simulink model "Boat_Sim"  (R2017a)
settings: Solver=VariableStepAuto  StartTime=0.0  StopTime=10.0  RelTol=1e-3
values from neighbouring files (symbols this model uses):
  J = zeros(2,2)    [ftle.m]
undefined symbols (not defined in the file or in its folder): K_omega, Kd, Km, Kv, M
libraries: simulink x2
settings Model: Creator=John  LastModifiedBy=John

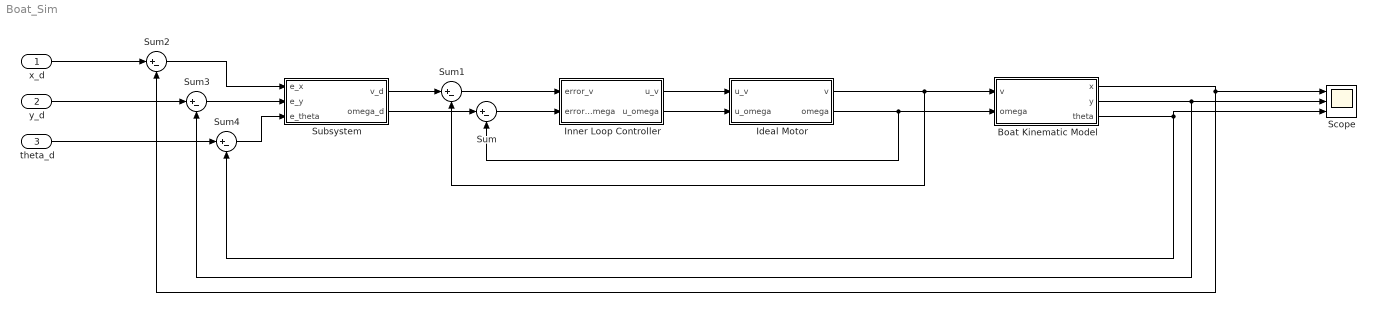
== system Boat_Sim ==
  x_d : Inport
  y_d : Inport  Port=2
  theta_d : Inport  Port=3
  Boat Kinematic Model : Subsystem
  Ideal Motor : Subsystem
  "Inner Loop Controller " : Subsystem
  Scope : Scope  NumInputPorts=3
  Subsystem : Subsystem
  Sum{,1..4} (5 alike) : Sum  Inputs=|+-
  wires:
  Boat Kinematic Model/1(x) -> Sum2/2, Scope/1
  Boat Kinematic Model/2(y) -> Sum3/2, Scope/2
  Boat Kinematic Model/3(theta) -> Sum4/2, Scope/3
  Ideal Motor/1(v) -> Sum1/2, Boat Kinematic Model/1(v)
  "Inner Loop Controller "/1(u_v) -> Ideal Motor/1(u_v)
  "Inner Loop Controller "/2(u_omega) -> Ideal Motor/2(u_omega)
  Sum/1 -> "Inner Loop Controller "/2(error_omega)
  Ideal Motor/2(omega) -> Sum/2, Boat Kinematic Model/2(omega)
  Sum1/1 -> "Inner Loop Controller "/1(error_v)
  x_d/1 -> Sum2/1
  y_d/1 -> Sum3/1
  theta_d/1 -> Sum4/1
  Sum2/1 -> Subsystem/1(e_x)
  Sum3/1 -> Subsystem/2(e_y)
  Sum4/1 -> Subsystem/3(e_theta)
  Subsystem/1(v_d) -> Sum1/1
  Subsystem/2(omega_d) -> Sum/1

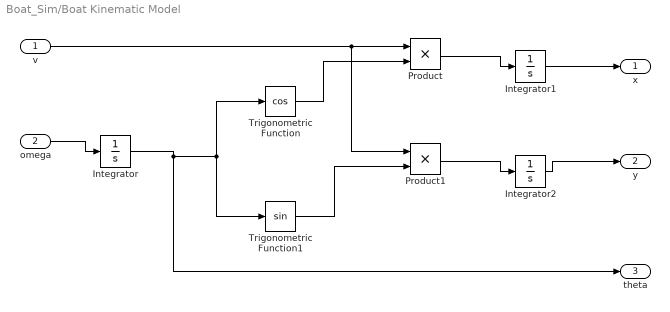
== system Boat_Sim/Boat Kinematic Model ==
  v : Inport
  omega : Inport  Port=2
  Integrator : Integrator
  Integrator1 : Integrator
  Integrator2 : Integrator
  Product : Product
  Product1 : Product
  Trigonometric Function : Trigonometry  Operator=cos
  Trigonometric Function1 : Trigonometry
  x : Outport
  y : Outport  Port=2
  theta : Outport  Port=3
  wires:
  Integrator1/1 -> x/1
  omega/1 -> Integrator/1
  Product1/1 -> Integrator2/1
  v/1 -> Product1/1, Product/1
  Trigonometric Function/1 -> Product/2
  Trigonometric Function1/1 -> Product1/2
  Product/1 -> Integrator1/1
  Integrator2/1 -> y/1
  Integrator/1 -> theta/1, Trigonometric Function1/1, Trigonometric Function/1
  ? -> ?

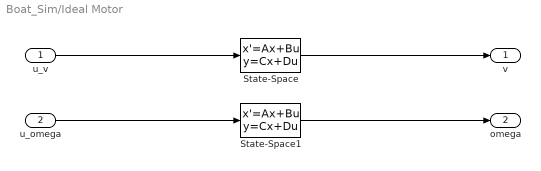
== system Boat_Sim/Ideal Motor ==
  u_v : Inport
  u_omega : Inport  Port=2
  State-Space : StateSpace  A=-Kv./M  B=Km./M  D=0  X0=0
  State-Space1 : StateSpace  A=-K_omega./J  B=Kd./J  D=0  X0=0  ContinuousStateAttributes='omega'
  v : Outport
  omega : Outport  Port=2
  wires:
  State-Space1/1 -> omega/1
  State-Space/1 -> v/1
  u_v/1 -> State-Space/1
  u_omega/1 -> State-Space1/1

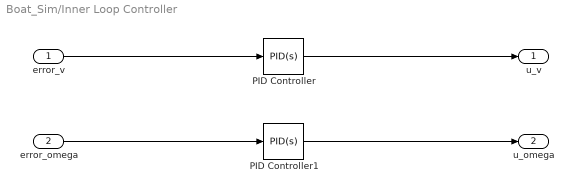
== system Boat_Sim/Inner Loop Controller  ==
  error_v : Inport
  error_omega : Inport  Port=2
  PID Controller : simulink/Continuous/PID Controller  Controller=PID  TimeDomain=Continuous-time  SampleTime=-1  IntegratorMethod=Forward Euler  FilterMethod=Forward Euler  Form=Parallel  UseFilter=on  ControllerParametersSource=internal  P=1  I=1  D=0  N=100  InitialConditionSource=internal  InitialConditionForIntegrator=0  InitialConditionForFilter=0  ExternalReset=none  LimitOutput=off  UpperSaturationLimit=inf  LowerSaturationLimit=-inf  LinearizeAsGain=on  AntiWindupMode=none  Kb=1  TrackingMode=off  Kt=1  PParamMin=[]  PParamMax=[]  IParamMin=[]  IParamMax=[]  DParamMin=[]  DParamMax=[]  NParamMin=[]  NParamMax=[]  KbParamMin=[]  KbParamMax=[]  KtParamMin=[]  KtParamMax=[]  POutMin=[]  POutMax=[]  IOutMin=[]  IOutMax=[]  DOutMin=[]  DOutMax=[]  NOutMin=[]  NOutMax=[]  KbOutMin=[]  KbOutMax=[]  KtOutMin=[]  KtOutMax=[]  IntegratorOutMin=[]  IntegratorOutMax=[]  FilterOutMin=[]  FilterOutMax=[]  SumOutMin=[]  SumOutMax=[]  SumI1OutMin=[]  SumI1OutMax=[]  SumI2OutMin=[]  SumI2OutMax=[]  SumI3OutMin=[]  SumI3OutMax=[]  SumDOutMin=[]  SumDOutMax=[]  SaturationOutMin=[]  SaturationOutMax=[]  IntegratorContinuousStateAttributes=''  IntegratorStateMustResolveToSignalObject=off  IntegratorRTWStateStorageClass=Auto  FilterContinuousStateAttributes=''  FilterStateMustResolveToSignalObject=off  FilterRTWStateStorageClass=Auto  DifferentiatorICPrevScaledInput=0  DifferentiatorOutMin=[]  DifferentiatorOutMax=[]  InitialConditionSetting=State (most efficient)
  PID Controller1 : simulink/Continuous/PID Controller  Controller=PID  TimeDomain=Continuous-time  SampleTime=-1  IntegratorMethod=Forward Euler  FilterMethod=Forward Euler  Form=Parallel  UseFilter=on  ControllerParametersSource=internal  P=1  I=1  D=0  N=100  InitialConditionSource=internal  InitialConditionForIntegrator=0  InitialConditionForFilter=0  ExternalReset=none  LimitOutput=off  UpperSaturationLimit=inf  LowerSaturationLimit=-inf  LinearizeAsGain=on  AntiWindupMode=none  Kb=1  TrackingMode=off  Kt=1  PParamMin=[]  PParamMax=[]  IParamMin=[]  IParamMax=[]  DParamMin=[]  DParamMax=[]  NParamMin=[]  NParamMax=[]  KbParamMin=[]  KbParamMax=[]  KtParamMin=[]  KtParamMax=[]  POutMin=[]  POutMax=[]  IOutMin=[]  IOutMax=[]  DOutMin=[]  DOutMax=[]  NOutMin=[]  NOutMax=[]  KbOutMin=[]  KbOutMax=[]  KtOutMin=[]  KtOutMax=[]  IntegratorOutMin=[]  IntegratorOutMax=[]  FilterOutMin=[]  FilterOutMax=[]  SumOutMin=[]  SumOutMax=[]  SumI1OutMin=[]  SumI1OutMax=[]  SumI2OutMin=[]  SumI2OutMax=[]  SumI3OutMin=[]  SumI3OutMax=[]  SumDOutMin=[]  SumDOutMax=[]  SaturationOutMin=[]  SaturationOutMax=[]  IntegratorContinuousStateAttributes=''  IntegratorStateMustResolveToSignalObject=off  IntegratorRTWStateStorageClass=Auto  FilterContinuousStateAttributes=''  FilterStateMustResolveToSignalObject=off  FilterRTWStateStorageClass=Auto  DifferentiatorICPrevScaledInput=0  DifferentiatorOutMin=[]  DifferentiatorOutMax=[]  InitialConditionSetting=State (most efficient)
  u_v : Outport
  u_omega : Outport  Port=2
  wires:
  error_omega/1 -> PID Controller1/1
  PID Controller1/1 -> u_omega/1
  error_v/1 -> PID Controller/1
  PID Controller/1 -> u_v/1

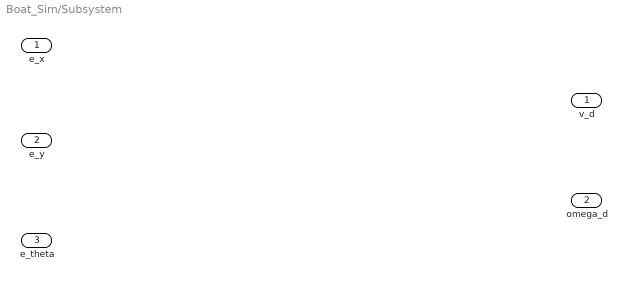
== system Boat_Sim/Subsystem ==
  e_x : Inport
  e_y : Inport  Port=2
  e_theta : Inport  Port=3
  v_d : Outport
  omega_d : Outport  Port=2
